simulink model "QlearningTest"  (R2015b)
settings: Solver=ode23t  SolverMode=SingleTasking  StartTime=0.0  StopTime=10  MaxStep=1e-5
InitFcn:
  | global R;
  | R = 2.875;
  | global L;
  | L = 0.00153;
  | SampleT = 1e-4;
  | R0 = 1.5;
  | L0 = 2e-3;
  | Beta1 = 10000;
  | Beta2 = 50000;
libraries: powerlib x1
Description:
  | Copyright 2008-2015 The MathWorks, Inc.
settings Model: ExtModeTrigMode=oneshot  ExtModeArmWhenConnect=off  ExtModeAutoUpdateStatusClock=off  Creator=MathWorks  LastModifiedBy=jxlllx
settings SolverCC: ZeroCrossAlgorithm=Adaptive  SolverResetMethod=Robust
settings DataIOCC: ExternalInput=[]  LimitDataPoints=off  SaveFormat=Array  SignalLoggingSaveFormat=ModelDataLogs  SaveOutput=off  SaveTime=off  SignalLoggingName=sigsOut
settings OptimizationCC: BlockReduction=off  BooleanDataType=off  ExpressionDepthLimit=2147483647  InitFltsAndDblsToZero=on  EfficientMapNaN2IntZero=off
settings DebuggingCC: UnderspecifiedInitializationDetection=Classic  MergeDetectMultiDrivingBlocksExec=none  CheckExecutionContextPreStartOutputMsg=on  CheckExecutionContextRuntimeOutputMsg=on  SignalResolutionControl=TryResolveAllWithWarning  MultiTaskDSMMsg=warning  MultiTaskCondExecSysMsg=none  SigSpecEnsureSampleTimeMsg=none  FcnCallInpInsideContextMsg=UseLocalSettings  StateNameClashWarn=warning
settings HardwareCC: ProdBitPerPointer=32  ProdLargestAtomicFloat=None  ProdIntDivRoundTo=Undefined  ProdEndianess=Unspecified  ProdWordSize=32  ProdHWDeviceType=32-bit Generic  TargetBitPerPointer=64  TargetLongLongMode=on  TargetIntDivRoundTo=Zero  TargetEndianess=LittleEndian  TargetWordSize=64  TargetHWDeviceType=MATLAB Host  ProdEqTarget=off
settings RTWCC: TargetLang=C++
settings GRTTargetCC: GeneratePreprocessorConditionals=Disable all  MultiInstanceERTCode=on  CodeInterfacePackaging=C++ class
settings ConfigComp: CovModelRefEnable=Off  CovSFcnEnable=off

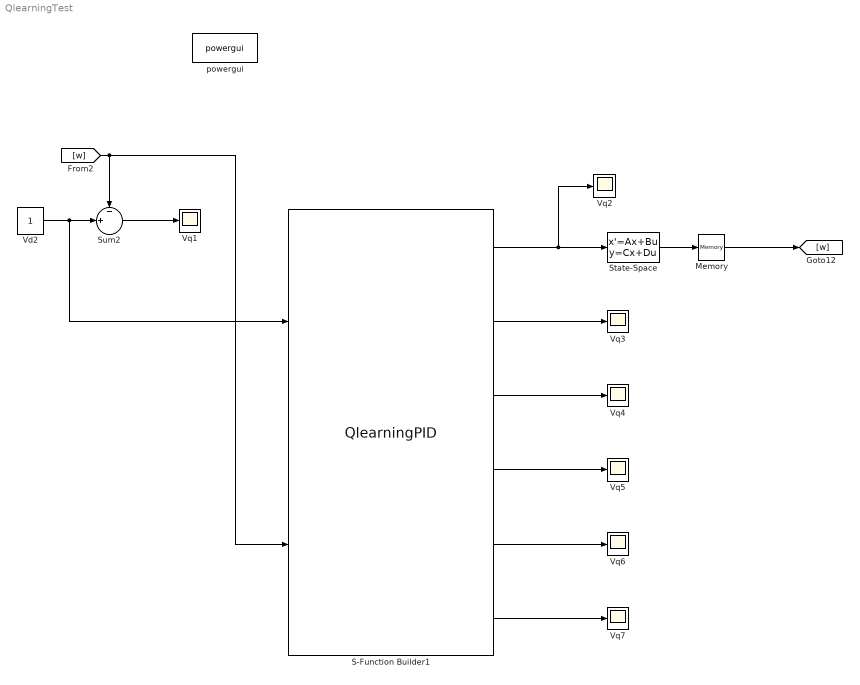
== system QlearningTest ==
  Memory : Memory
  S-Function Builder1 : S-Function  InitFcn=try, set_param(gcb,'FunctionName','QlearningPID'), end  FunctionName=QlearningPID  SFunctionModules=QlearningPID_wrapper PID RL_Brain  SFunctionDeploymentMode=off  EnableBusSupport=off  mask(S-Function Builder){}
      mask help: Simulink:masks:SFunctionBuilder_MD
      mask init:
      | val = [[.9  0.75 0.75 1 1 .9 .9 1]',[1 1 0.75 0.75 .9 .9 1 .9]'];try , sys = get_param(gcb,'SfunBuilderFcnName');if isempty(sys), sys = get_param(gcb,'FunctionName'); end,catch, sys = get_param(gcb,'FunctionName'); end
      settings: CopyFcn=set_param(gcbh,'LinkStatus','none')  PreSaveFcn=try, set_param(gcb,'FunctionName','QlearningPID'), end  OpenFcn=sfunctionwizard(gcbh)
      mask Display: plot(val(:,1),val(:,2)),disp(sys), port_label('input',1,'Ref'), port_label('input',2,'Out'), port_label('output',1,'u0'), port_label('output',2,'ActionNumOut'), port_label('output',3,'StateSeqAllOut'), port_label('output',4,'errorStateOut'), port_label('output',5,'errorIntegStateOut'), port_label('output',6,'errorDiffStateOut')
  State-Space : StateSpace  A=-3  D=0  X0=0
  Sum2 : Sum  Inputs=-|+||
  Vd2 : Constant
  Vq{1..7} (7 alike) : Scope
  powergui : powerlib/powergui  SimulationMode=Continuous  SolverType=Tustin  SampleTime=0  frequency=60  SPID=on  DisableSnubberDevices=off  DisableRonSwitches=off  DisableVfSwitches=off  SwTol=0  DisplayEquations=off  Interpol=off  ExternalGateDelay=off  methode=off  Ts=0  FunctionMessages=off  echomessages=off  HookPort=off  EnableUseOfTLC=off  x0status=blocks  frequencyindice=0  Pbase=100e6  ErrMax=1e-4  Iterations=50  UnitsV=kV  UnitsW=MW  buscounter=0  RestoreLinks=warning  ResistiveCurrentMeasurement=off  Frange=[0:2:500]  Ylog=off  Xlog=on  ShowGrid=off  save=off  variable=ZData  structure=0  ZoomFFT=on  StartTime=0.0  cycles=1  DisplayStyle=1  fundamental=60  FreqAxis=off  MaxFrequency=1000  frequencyindicesteady=1  RmsSteady=1  display=off
  wires:
  Vd2/1 -> Sum2/2, S-Function Builder1/1
  [w] -> Sum2/1, S-Function Builder1/2
  Sum2/1 -> Vq1/1
  Memory/1 -> [w]
  State-Space/1 -> Memory/1
  S-Function Builder1/1 -> Vq2/1, State-Space/1
  S-Function Builder1/2 -> Vq3/1
  S-Function Builder1/3 -> Vq4/1
  S-Function Builder1/4 -> Vq5/1
  S-Function Builder1/5 -> Vq6/1
  S-Function Builder1/6 -> Vq7/1
